simulink model "UAV"  (R2016a)
settings: Solver=ode4  StartTime=0.0  StopTime=10.0  FixedStep=0.001  RelTol=1e-3
settings Model: Creator=Administrator  LastModifiedBy=Administrator

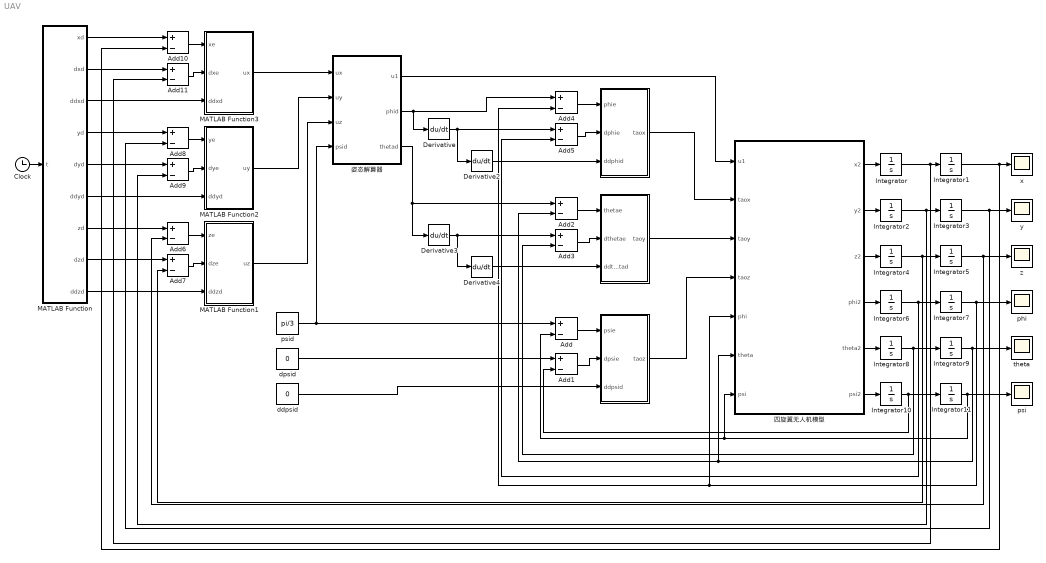
== system UAV ==
  " " : MATLAB Function  TreatAsAtomicUnit=on
  " " : MATLAB Function  TreatAsAtomicUnit=on
  " " : MATLAB Function  TreatAsAtomicUnit=on
  Add{,1..11} (12 alike) : Sum  Inputs=+-
  Clock : Clock
  Derivative{,2..4} (4 alike) : Derivative
  Integrator{,1..11} (12 alike) : Integrator
  MATLAB Function : MATLAB Function  TreatAsAtomicUnit=on
  MATLAB Function1 : MATLAB Function  TreatAsAtomicUnit=on
  MATLAB Function2 : MATLAB Function  TreatAsAtomicUnit=on
  MATLAB Function3 : MATLAB Function  TreatAsAtomicUnit=on
  ddpsid : Constant  Value=0
  dpsid : Constant  Value=0
  phi : Scope
  psi : Scope
  psid : Constant  Value=pi/3
  theta : Scope
  x : Scope
  y : Scope
  z : Scope
  四旋翼无人机模型 : MATLAB Function  TreatAsAtomicUnit=on
  姿态解算器 : MATLAB Function  TreatAsAtomicUnit=on
  wires:
  四旋翼无人机模型/1(x2) -> Integrator/1
  四旋翼无人机模型/2(y2) -> Integrator2/1
  四旋翼无人机模型/3(z2) -> Integrator4/1
  Integrator5/1 -> Add6/2, z/1
  四旋翼无人机模型/4(phi2) -> Integrator6/1
  四旋翼无人机模型/5(theta2) -> Integrator8/1
  四旋翼无人机模型/6(psi2) -> Integrator10/1
  Integrator10/1 -> Integrator11/1, Add1/2
  Integrator11/1 -> psi/1, Add/2, 四旋翼无人机模型/7(psi)
  psid/1 -> 姿态解算器/4(psid), Add/1
  dpsid/1 -> Add1/1
  " "/1(taoz) -> 四旋翼无人机模型/4(taoz)
  Add1/1 -> " "/2(dpsie)
  Add/1 -> " "/1(psie)
  ddpsid/1 -> " "/3(ddpsid)
  Integrator8/1 -> Integrator9/1, Add3/2
  Integrator9/1 -> Add2/2, 四旋翼无人机模型/6(theta), theta/1
  姿态解算器/3(thetad) -> Derivative3/1, Add2/1
  " "/1(taoy) -> 四旋翼无人机模型/3(taoy)
  Add3/1 -> " "/2(dthetae)
  Add2/1 -> " "/1(thetae)
  Derivative4/1 -> " "/3(ddthetad)
  Integrator6/1 -> Integrator7/1, Add5/2
  Integrator7/1 -> Add4/2, 四旋翼无人机模型/5(phi), phi/1
  Derivative/1 -> Derivative2/1, Add5/1
  " "/1(taox) -> 四旋翼无人机模型/2(taox)
  Add5/1 -> " "/2(dphie)
  Add4/1 -> " "/1(phie)
  Derivative2/1 -> " "/3(ddphid)
  姿态解算器/1(u1) -> 四旋翼无人机模型/1(u1)
  姿态解算器/2(phid) -> Add4/1, Derivative/1
  Derivative3/1 -> Derivative4/1, Add3/1
  Clock/1 -> MATLAB Function/1(t)
  MATLAB Function/7(zd) -> Add6/1
  Add6/1 -> MATLAB Function1/1(ze)
  Add7/1 -> MATLAB Function1/2(dze)
  MATLAB Function/8(dzd) -> Add7/1
  Integrator4/1 -> Integrator5/1, Add7/2
  MATLAB Function/9(ddzd) -> MATLAB Function1/3(ddzd)
  MATLAB Function1/1(uz) -> 姿态解算器/3(uz)
  Integrator3/1 -> Add8/2, y/1
  MATLAB Function/4(yd) -> Add8/1
  Add8/1 -> MATLAB Function2/1(ye)
  Add9/1 -> MATLAB Function2/2(dye)
  MATLAB Function/5(dyd) -> Add9/1
  Integrator2/1 -> Add9/2, Integrator3/1
  MATLAB Function/6(ddyd) -> MATLAB Function2/3(ddyd)
  MATLAB Function2/1(uy) -> 姿态解算器/2(uy)
  Integrator1/1 -> Add10/2, x/1
  MATLAB Function/1(xd) -> Add10/1
  Add10/1 -> MATLAB Function3/1(xe)
  Add11/1 -> MATLAB Function3/2(dxe)
  MATLAB Function/2(dxd) -> Add11/1
  Integrator/1 -> Add11/2, Integrator1/1
  MATLAB Function3/1(ux) -> 姿态解算器/1(ux)
  MATLAB Function/3(ddxd) -> MATLAB Function3/3(ddxd)

== matlab function UAV/  ==
  data: psie input; taoz output; dpsie input; ddpsid input
function taoz = fcn(psie, dpsie, ddpsid)
%#codegen
%%定义参数
Jzz = 0.0186;
kppsi = 36;
kdpsi = 12;

%%控制率
taoz = Jzz*(kppsi*psie+kdpsi*dpsie+ddpsid);
end

== matlab function UAV/四旋翼无人机模型 ==
  data: u1 input; x2 output; taox input; taoy input; taoz input; phi input; theta input; psi input; y2 output; z2 output; phi2 output; theta2 output; psi2 output
function [x2, y2, z2, phi2, theta2, psi2]= fcn(u1, taox, taoy, taoz, phi, theta, psi)
%#codegen
%%四旋翼无人机相关参数
m = 1.023 ;
g = 9.81;
Jxx = 0.0095 ;
Jyy = 0.0095 ;
Jzz = 0.0186 ;
%%搭建无人机位置环模型
x2 = u1/m + (sin(phi)*sin(psi)+cos(phi)*sin(theta)*cos(psi));
y2 = u1/m + (cos(phi)*sin(theta)*sin(psi)-sin(phi)*cos(psi));
z2 = u1/m*cos(phi)*cos(theta)-g;

%%姿态环模型
phi2 = taox/Jxx;
theta2 = taoy/Jyy;
psi2 = taoz/Jzz;

end

== matlab function UAV/  ==
  data: thetae input; taoy output; dthetae input; ddthetad input
function taoy = fcn(thetae, dthetae, ddthetad)
%#codegen
%%定义参数
Jyy = 0.0095;
kptheta = 169;
kdtheta = 26;

%%控制率
taoy = Jyy*(kptheta*thetae+kdtheta*dthetae+ddthetad);
end

== matlab function UAV/  ==
  data: phie input; taox output; dphie input; ddphid input
function taox = fcn(phie, dphie, ddphid)
%#codegen
%%定义参数
Jxx = 0.0095;
kpphi = 169;
kdphi = 26;

%%控制率
taox = Jxx*(kpphi*phie+kdphi*dphie+ddphid);
end

== matlab function UAV/姿态解算器 ==
  data: ux input; u1 output; uy input; uz input; phid output; thetad output; psid input
function [u1, phid, thetad] = fcn(ux, uy, uz, psid)
%#codegen
%
thetad = atan((cos(psid)*ux+sin(psid)*uy)/uz);
phid = atan((sin(psid)*ux-cos(psid)*uy)/(sqrt((cos(psid)*ux+sin(psid)*uy)^2)+uz^2));
u1 = uz/(cos(phid)*cos(thetad));

end

== matlab function UAV/MATLAB Function ==
  data: t input; xd output; dxd output; ddxd output; yd output; dyd output; ddyd output; zd output; dzd output; ddzd output
function [xd, dxd, ddxd, yd, dyd, ddyd, zd, dzd, ddzd] = fcn(t)
%#codegen
xd = cos(0.5*t);
dxd = -0.5*sin(0.5*t);
ddxd = -0.25*cos(0.5*t);

yd = sin(0.5*t);
dyd = 0.5*cos(0.5*t);
ddyd = -0.25*sin(0.5*t);

zd = 1;
dzd = 0;
ddzd = 0;

end

== matlab function UAV/MATLAB Function1 ==
  data: ze input; uz output; dze input; ddzd input
function uz = fcn(ze, dze, ddzd)
%%相关参数
m = 1.023;
g = 9.81;
kpz = 25;
kdz = 10;

%%控制率
uz = m*(kpz*ze+kdz*dze+g+ddzd);
end

== matlab function UAV/MATLAB Function2 ==
  data: ye input; uy output; dye input; ddyd input
function uy = fcn(ye, dye, ddyd)
%%相关参数
m = 1.023;
g = 9.81;
kpy = 10/3;
kdy = 25/9;

%%控制率
uy = m*(kpy*ye+kdy*dye+ddyd);
end

== matlab function UAV/MATLAB Function3 ==
  data: xe input; ux output; dxe input; ddxd input
function ux = fcn(xe, dxe, ddxd)
%%相关参数
m = 1.023;
kpx = 10/3;
kdx = 25/9;

%%控制率
ux = m*(kpx*xe+kdx*dxe+ddxd);
